simulink model "sgMdl_CAN_ParsingAndMapping"  (R2024b)
settings: Solver=FixedStepAuto  StartTime=0.0  StopTime=inf  RelTol=1e-3  EnableMultiTasking=on
model workspace (MAT data in the model file):
  mdlWSDbList = []
  mdlWSDbcList = "canConnectivityForVehicle.dbc"
undefined symbols (not defined in the file): DiscIntNeverNeededParam, Down, IO602, Pull
libraries: simulink x3, speedgoatlib_IO602_4 x1
Description:
  | CAN - Working with the DB Parser
settings Model: ModifiedByFormat=Speedgoat  Creator=Speedgoat  LastModifiedBy=Speedgoat
settings SolverCC: ConcurrentTasks=on  AlgebraicLoopSolver=TrustRegion  PositivePriorityOrder=on  InsertRTBMode=Never (minimum delay)
settings DataIOCC: SaveFormat=Array  SignalLoggingName=logsOut
settings OptimizationCC: BlockReduction=off  BooleanDataType=off  OptimizeBlockIOStorage=off  BufferReuse=off  ReuseModelBlockBuffer=off  GlobalBufferReuse=off  ExpressionFolding=off  LocalBlockOutputs=off  InitFltsAndDblsToZero=on  OptimizeDataStoreBuffers=off  BusAssignmentInplaceUpdate=off
settings DebuggingCC: SaveWithParameterizedLinksMsg=none  UnderspecifiedInitializationDetection=Classic  MergeDetectMultiDrivingBlocksExec=none  CheckExecutionContextPreStartOutputMsg=on  SignalResolutionControl=TryResolveAllWithWarning  TasksWithSamePriorityMsg=none  UnconnectedInputMsg=warning  UnconnectedOutputMsg=warning  UnconnectedLineMsg=warning  SFUnexpectedBacktrackingDiag=warning  SFNoUnconditionalDefaultTransitionDiag=warning  SFExecutionAtInitializationDiag=none  ArithmeticOperatorsInVariantConditions=warning
settings HardwareCC: ProdBitPerLong=64  ProdLongLongMode=on  ProdHWDeviceType=Intel->x86-64 (Linux 64)
settings ModelReferenceCC: EnableRefExpFcnMdlSchedulingChecks=on  PropagateSignalLabelsOutOfModel=off
settings SFSimCC: SimUseLocalCustomCode=off  SimTargetLang=C++
settings RTWCC: Description=Speedgoat Real-Time Target Machine  SystemTargetFile=speedgoat.tlc  TemplateMakefile=slrealtime_default_tmf  RTWUseLocalCustomCode=off  Toolchain=Simulink Real-Time Toolchain  BuildConfiguration=Faster Runs  TargetLang=C++  GPUComputeCapability=3.5  DLArmComputeVersion=19.05
settings CodeAppCC: StateflowObjectComments=on
settings SimulinkRealTimeTargetCC: SubcomponentCodeInterfacePackaging=Reusable function  MATLABClassNameForMDSCustomization=Simulink.SoftwareTarget.GRTCustomization  InstructionSetFMA=off  LogToMDFFile=off  SLRTFileLogMaxRuns=10
settings ConfigComp: CovMetricSettings=dw  CovSaveCumulativeToWorkspaceVar=on  CovSaveSingleToWorkspaceVar=on  CovExternalEMLEnable=off  CovSFcnEnable=off  CovBoundaryAbsTol=1.0e-5

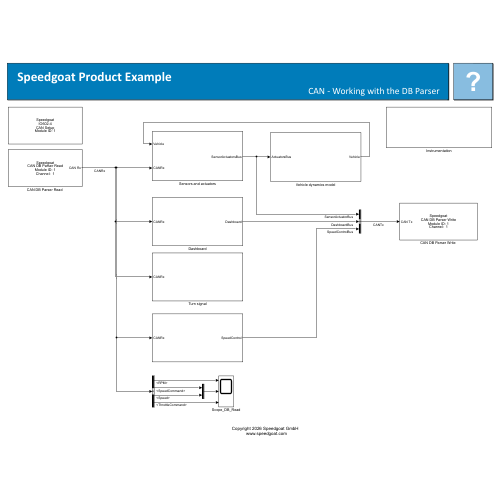
[thumbnail: Simulink's stored preview of the top-level diagram]
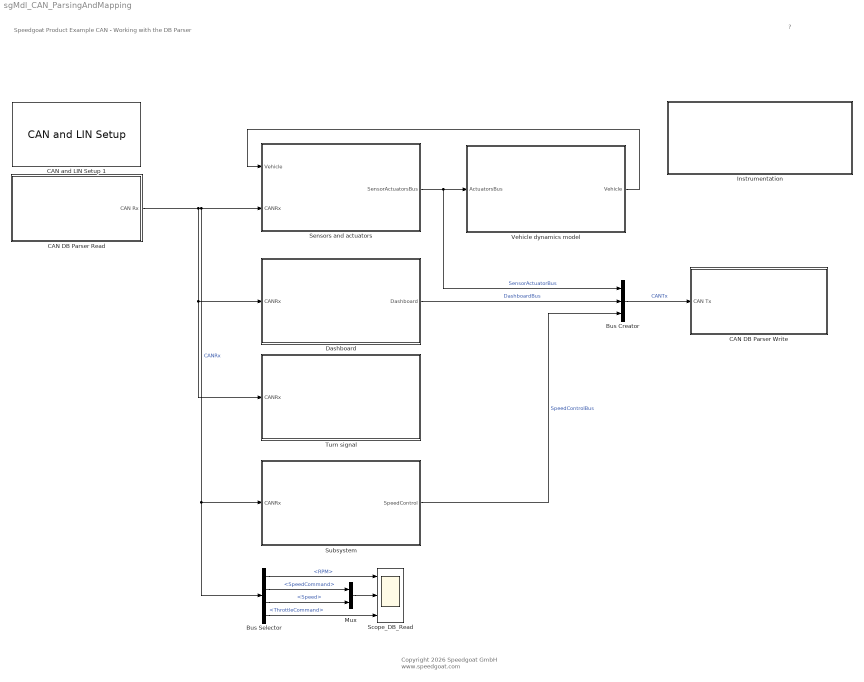
== system sgMdl_CAN_ParsingAndMapping ==
  note: Speedgoat Product Example
      | CAN - Working with the DB Parser
  note: ?
  note: Copyright 2026 Speedgoat GmbH
      |  www.speedgoat.com
  Bus Creator : BusCreator  Inputs=3
  Bus Selector : BusSelector  OutputSignals=ID2048_RPMMessage.RPM,ID1024_SpeedCommandMessage.SpeedCommand,ID256_SpeedMessage.Speed,ID96_ThrottleCommandMessage.ThrottleCommand
  "CAN DB Parser Read " : Subsystem
      settings: OpenFcn=sg_can.OpenFcnRead;
      mask Help: eval('sg.utils.help.show(''io_main/refentry_ref_can_ofa_parsing_read'');')
      mask Display: disp('Speedgoat\nCAN DB Parser Read\nModule ID: 1\nChannel:  1');
  "CAN DB Parser Write " : Subsystem
      settings: OpenFcn=sg_can.OpenFcnWrite;
      mask Help: eval('sg.utils.help.show(''io_main/refentry_ref_can_ofa_parsing_write'');')
      mask Display: disp('Speedgoat\nCAN DB Parser Write\nModule ID: 1\nChannel:  1');
  CAN and LIN Setup 1 : speedgoatlib_IO602_4/CAN and LIN Setup   moduleInitValues="[6022     1     1    -1    -1]"  id=1  moduleType=IO602-2  pciSlot=-1  canChn1=CAN (HS)  canChn2=CAN (HS)  canChn3=Disabled  canChn4=Disabled  linChn1=Disabled  linChn2=Disabled  canInitStructArray=[]  canTermStructArray=[]  gpioChnx=Disabled  canChn1InitValues="[2   2   8   1  16   3  19   2   2   5   2   0]"  arbBdrChn1=500 kBaud  clockDividerChn1=Enable  arbManBdrChn1=[8,1,16,3]  fdBdrChn1=5.0 MBaud  fdManBdrChn1=[2,2,5,2]  termResistor1=off  canChn2InitValues="[2   2   8   1  16   3  19   2   2   5   2   0]"  arbBdrChn2=500 kBaud  clockDividerChn2=Enable  arbManBdrChn2=[8,1,16,3]  fdBdrChn2=5.0 MBaud  fdManBdrChn2=[2,2,5,2]  termResistor2=off  canChn3InitValues="[1   0   2   8  31   8  19   2   2   5   2   0]"  arbBdrChn3=1.0 MBaud  clockDividerChn3=Enable  arbManBdrChn3=[2,8,31,8]  fdBdrChn3=5.0 MBaud  fdManBdrChn3=[2,2,5,2]  termResistor3=off  canChn4InitValues="[1   0   2   8  31   8  19   2   2   5   2   0]"  arbBdrChn4=1.0 MBaud  clockDividerChn4=Enable  arbManBdrChn4=[2,8,31,8]  fdBdrChn4=5.0 MBaud  fdManBdrChn4=[2,2,5,2]  termResistor4=off  linChn1InitValues="[0  9600]"  linBtrChn1=9600  linChn2InitValues="[0  9600]"  linBtrChn2=9600  doInitTermStruct="[0  5  0  0  0]"  parDoChannels=[1 2]  parDoVoltage=5  parDoInitValues=0  parDoReset=1  parNumOfDoS=0  parDiChannels=[3 4]  parDiVoltage=5  parDiPull=Pull-Down
      settings: LibrarySourceBlock=speedgoatlib_IO602_IO691/CAN and LIN Setup  SourceProductName=IO602-4
  Dashboard : Subsystem
  Instrumentation : Subsystem
  Mux : Mux  Inputs=2
  Scope_DB_Read : Scope  NumInputPorts=3
  Sensors and actuators : Subsystem
  Subsystem : Subsystem
  Turn signal : Subsystem
  Vehicle dynamics model : Subsystem
  wires:
  Vehicle dynamics model/1(Vehicle) -> Sensors and actuators/1(Vehicle)
  Sensors and actuators/1(SensorActuatorsBus) -> Bus Creator/1, Vehicle dynamics model/1(ActuatorsBus)  "SensorActuatorBus"
  Bus Creator/1 -> "CAN DB Parser Write "/1(CAN Tx)  "CANTx"
  Dashboard/1(Dashboard) -> Bus Creator/2  "DashboardBus"
  Subsystem/1(SpeedControl) -> Bus Creator/3  "SpeedControlBus"
  Mux/1 -> Scope_DB_Read/2
  Bus Selector/3 -> Mux/2  "<Speed>"
  Bus Selector/2 -> Mux/1  "<SpeedCommand>"
  "CAN DB Parser Read "/1(CAN Rx) -> Turn signal/1(CANRx), Dashboard/1(CANRx), Bus Selector/1, Subsystem/1(CANRx), Sensors and actuators/2(CANRx)  "CANRx"
  Bus Selector/1 -> Scope_DB_Read/1  "<RPM>"
  Bus Selector/4 -> Scope_DB_Read/3  "<ThrottleCommand>"

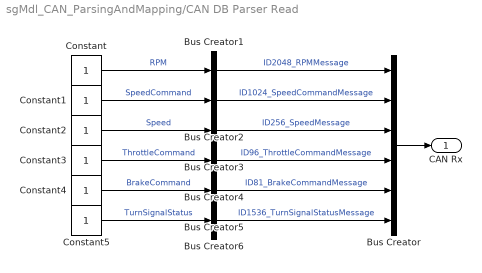
== system sgMdl_CAN_ParsingAndMapping/CAN DB Parser Read  ==
  Bus Creator : BusCreator  Inputs=6
  Bus Creator{1..6} (6 alike) : BusCreator  Inputs=1
  Constant{,1..5} (6 alike) : Constant  SampleTime=-1
  CAN Rx : Outport
  wires:
  Bus Creator4/1 -> Bus Creator/4  "ID96_ThrottleCommandMessage"
  Bus Creator1/1 -> Bus Creator/1  "ID2048_RPMMessage"
  Constant2/1 -> Bus Creator3/1  "Speed"
  Bus Creator2/1 -> Bus Creator/2  "ID1024_SpeedCommandMessage"
  Bus Creator5/1 -> Bus Creator/5  "ID81_BrakeCommandMessage"
  Constant5/1 -> Bus Creator6/1  "TurnSignalStatus"
  Constant4/1 -> Bus Creator5/1  "BrakeCommand"
  Constant1/1 -> Bus Creator2/1  "SpeedCommand"
  Constant3/1 -> Bus Creator4/1  "ThrottleCommand"
  Bus Creator/1 -> CAN Rx/1
  Bus Creator3/1 -> Bus Creator/3  "ID256_SpeedMessage"
  Constant/1 -> Bus Creator1/1  "RPM"
  Bus Creator6/1 -> Bus Creator/6  "ID1536_TurnSignalStatusMessage"

== system sgMdl_CAN_ParsingAndMapping/CAN DB Parser Write  ==
  CAN Tx : Inport
  Terminator : Terminator
  wires:
  CAN Tx/1 -> Terminator/1

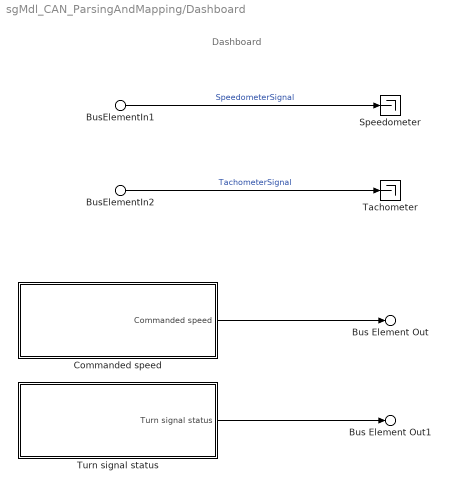
== system sgMdl_CAN_ParsingAndMapping/Dashboard ==
  note: Dashboard
  BusElementIn1 : Inport  PortName=CANRx  Element=ID256_SpeedMessage.Speed
  BusElementIn2 : Inport  PortName=CANRx  Element=ID2048_RPMMessage.RPM
  Commanded speed : Subsystem
  Speedometer : Terminator
  Tachometer : Terminator
  Turn signal status : Subsystem
  Bus Element Out : Outport  PortName=Dashboard  Element=SpeedComand
  Bus Element Out1 : Outport  PortName=Dashboard  Element=TurnSignalStatus
  wires:
  BusElementIn2/1 -> Tachometer/1  "TachometerSignal"
  BusElementIn1/1 -> Speedometer/1  "SpeedometerSignal"
  Commanded speed/1(Commanded speed) -> Bus Element Out/1
  Turn signal status/1(Turn signal status) -> Bus Element Out1/1

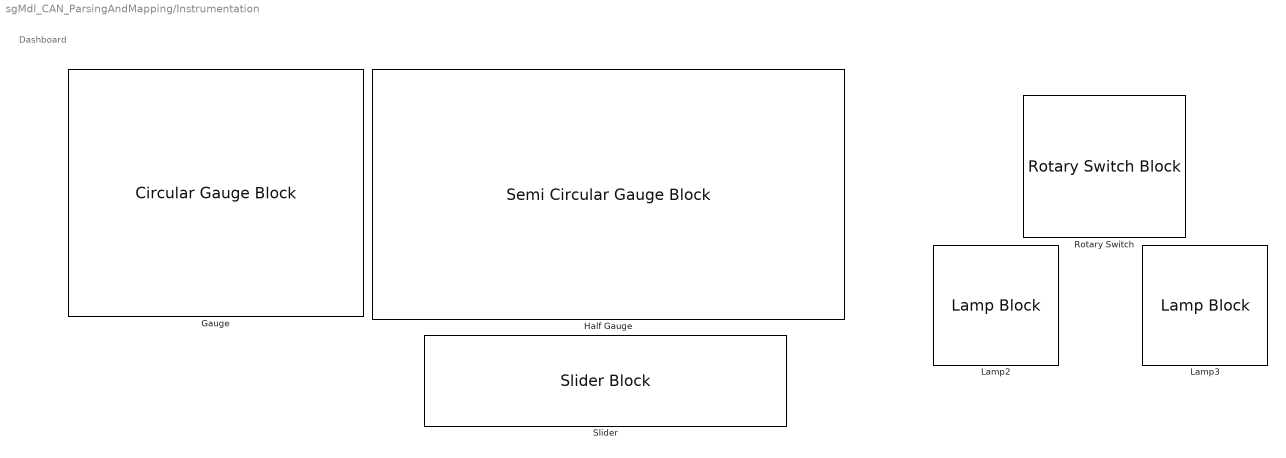
== system sgMdl_CAN_ParsingAndMapping/Instrumentation ==
  note: Dashboard
  Gauge : CircularGaugeBlock  TickInterval=10
  Half Gauge : SemiCircularGaugeBlock  ScaleMax=9000  TickInterval=1000
  Lamp2 : LampBlock
  Lamp3 : LampBlock
  Rotary Switch : RotarySwitchBlock
      settings: Values={{'Left', 'Off', 'Right'}, [1 2 3]}
  Slider : SliderBlock

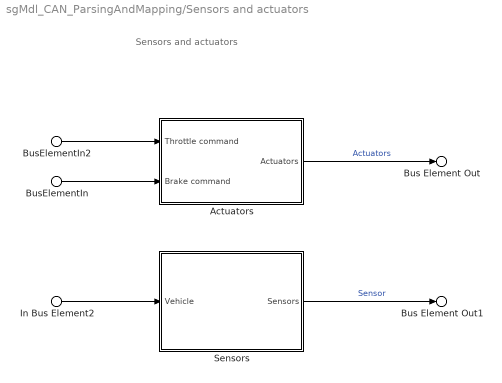
== system sgMdl_CAN_ParsingAndMapping/Sensors and actuators ==
  note: Sensors and actuators
  In Bus Element2 : Inport  PortName=Vehicle
  BusElementIn2 : Inport  Port=2  PortName=CANRx  Element=ID96_ThrottleCommandMessage.ThrottleCommand
  BusElementIn : Inport  Port=2  PortName=CANRx  Element=ID81_BrakeCommandMessage.BrakeCommand
  Actuators : Subsystem
  Sensors : Subsystem
  Bus Element Out : Outport  PortName=SensorActuatorsBus  Element=Actuators
  Bus Element Out1 : Outport  PortName=SensorActuatorsBus  Element=Sensors
  wires:
  Actuators/1(Actuators) -> Bus Element Out/1  "Actuators"
  Sensors/1(Sensors) -> Bus Element Out1/1  "Sensor"
  BusElementIn2/1 -> Actuators/1(Throttle command)
  BusElementIn/1 -> Actuators/2(Brake command)
  In Bus Element2/1 -> Sensors/1(Vehicle)

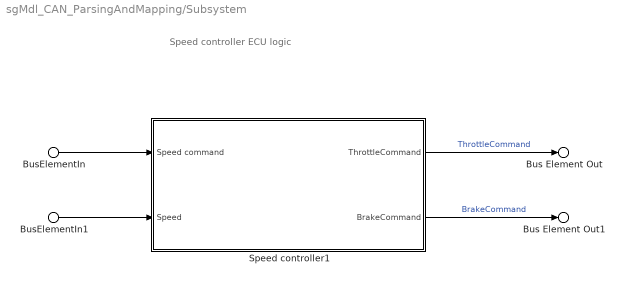
== system sgMdl_CAN_ParsingAndMapping/Subsystem ==
  note: Speed controller ECU logic
  BusElementIn : Inport  PortName=CANRx  Element=ID1024_SpeedCommandMessage.SpeedCommand
  BusElementIn1 : Inport  PortName=CANRx  Element=ID256_SpeedMessage.Speed
  Speed controller1 : Subsystem
  Bus Element Out : Outport  PortName=SpeedControl  Element=ThrottleCommand
  Bus Element Out1 : Outport  PortName=SpeedControl  Element=BrakeCommand
  wires:
  BusElementIn/1 -> Speed controller1/1(Speed command)
  BusElementIn1/1 -> Speed controller1/2(Speed)
  Speed controller1/1(ThrottleCommand) -> Bus Element Out/1  "ThrottleCommand"
  Speed controller1/2(BrakeCommand) -> Bus Element Out1/1  "BrakeCommand"

== system sgMdl_CAN_ParsingAndMapping/Turn signal ==
  note: Turn signal ECU logic
  BusElementIn : Inport  PortName=CANRx  Element=ID1536_TurnSignalStatusMessage.TurnSignalStatus
  Left turn signal : Terminator
  Right turn signal : Terminator
  Turn signal logic : Subsystem
  wires:
  Turn signal logic/1(Left turn signal interface) -> Left turn signal/1  "LeftTurnSignal"
  Turn signal logic/2(Right turn signal interface) -> Right turn signal/1  "RightTurnSignal"
  BusElementIn/1 -> Turn signal logic/1(Turn signal status)

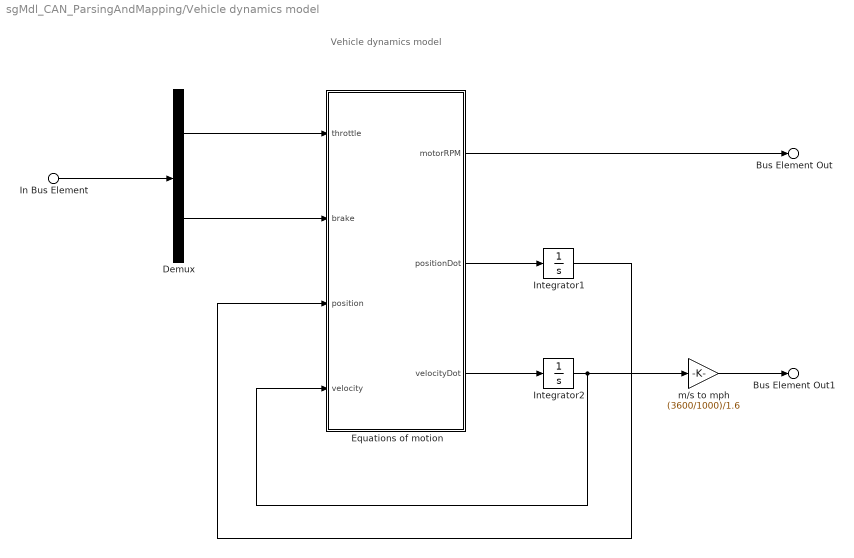
== system sgMdl_CAN_ParsingAndMapping/Vehicle dynamics model ==
  note: Vehicle dynamics model
  In Bus Element : Inport  PortName=ActuatorsBus  Element=Actuators.Control
  Demux : Demux  Outputs=2
  Equations of motion : Subsystem
  Integrator1 : Integrator
  Integrator2 : Integrator
  m/s to mph : Gain  Gain=(3600/1000)/1.6
  Bus Element Out : Outport  PortName=Vehicle  Element=motorRPM
  Bus Element Out1 : Outport  PortName=Vehicle  Element=Velocity
  wires:
  Demux/1 -> Equations of motion/1(throttle)
  Equations of motion/2(positionDot) -> Integrator1/1
  Equations of motion/3(velocityDot) -> Integrator2/1
  Integrator2/1 -> Equations of motion/4(velocity), m/s to mph/1
  Integrator1/1 -> Equations of motion/3(position)
  Demux/2 -> Equations of motion/2(brake)
  Equations of motion/1(motorRPM) -> Bus Element Out/1
  In Bus Element/1 -> Demux/1
  m/s to mph/1 -> Bus Element Out1/1

== system sgMdl_CAN_ParsingAndMapping/Dashboard/Commanded speed ==
  note: Commanded speed
  Speed command : Constant  Value=33.01438748428551  OutDataTypeStr=double  SampleTime=Inf
  Zero-Order Hold : ZeroOrderHold  SampleTime=-1
  Commanded speed : Outport  VectorParamsAs1DForOutWhenUnconnected=off
  wires:
  Speed command/1 -> Zero-Order Hold/1
  Zero-Order Hold/1 -> Commanded speed/1

== system sgMdl_CAN_ParsingAndMapping/Dashboard/Turn signal status ==
  note: Turn signal status
  Turn signal : Constant  Value=2  OutDataTypeStr=double
  Zero-Order Hold : ZeroOrderHold  SampleTime=-1
  Turn signal status : Outport  VectorParamsAs1DForOutWhenUnconnected=off
  wires:
  Turn signal/1 -> Zero-Order Hold/1
  Zero-Order Hold/1 -> Turn signal status/1

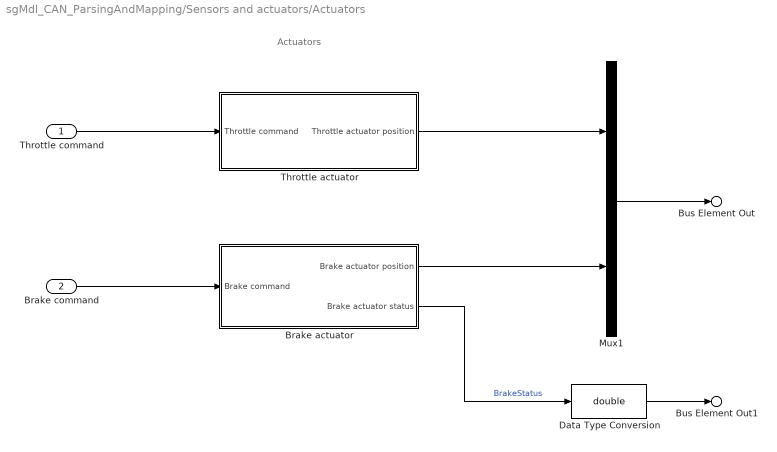
== system sgMdl_CAN_ParsingAndMapping/Sensors and actuators/Actuators ==
  note: Actuators
  Throttle command : Inport
  Brake command : Inport  Port=2
  Brake actuator : Subsystem
  Data Type Conversion : DataTypeConversion  OutDataTypeStr=double  SaturateOnIntegerOverflow=off  RndMeth=Floor
  Mux1 : Mux  Inputs=2
  Throttle actuator : Subsystem
  Bus Element Out : Outport  PortName=Actuators  Element=Control
  Bus Element Out1 : Outport  PortName=Actuators  Element=BrakeStatus
  wires:
  Brake actuator/1(Brake actuator position) -> Mux1/2
  Throttle actuator/1(Throttle actuator position) -> Mux1/1
  Brake command/1 -> Brake actuator/1(Brake command)
  Throttle command/1 -> Throttle actuator/1(Throttle command)
  Data Type Conversion/1 -> Bus Element Out1/1
  Brake actuator/2(Brake actuator status) -> Data Type Conversion/1  "BrakeStatus"
  Mux1/1 -> Bus Element Out/1

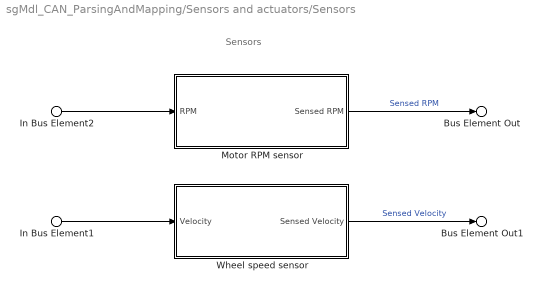
== system sgMdl_CAN_ParsingAndMapping/Sensors and actuators/Sensors ==
  note: Sensors
  In Bus Element2 : Inport  PortName=Vehicle  Element=motorRPM
  In Bus Element1 : Inport  PortName=Vehicle  Element=Velocity
  Motor RPM sensor : Subsystem
  Wheel speed sensor : Subsystem
  Bus Element Out : Outport  PortName=Sensors  Element=RPM
  Bus Element Out1 : Outport  PortName=Sensors  Element=Speed
  wires:
  In Bus Element2/1 -> Motor RPM sensor/1(RPM)
  In Bus Element1/1 -> Wheel speed sensor/1(Velocity)
  Wheel speed sensor/1(Sensed Velocity) -> Bus Element Out1/1  "Sensed Velocity"
  Motor RPM sensor/1(Sensed RPM) -> Bus Element Out/1  "Sensed RPM"

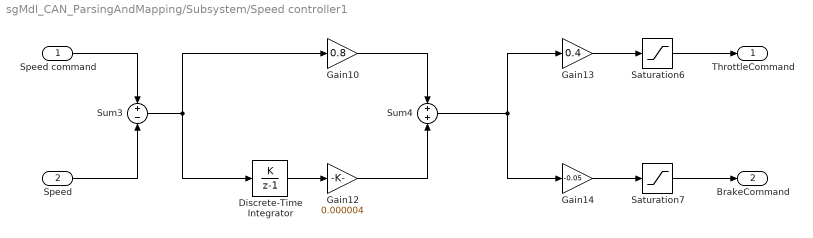
== system sgMdl_CAN_ParsingAndMapping/Subsystem/Speed controller1 ==
  Speed command : Inport
  Speed : Inport  Port=2
  Discrete-Time Integrator : DiscreteIntegrator  IntegratorMethod=Accumulation: Forward Euler  SampleTime=-1  ICPrevOutput=DiscIntNeverNeededParam  ICPrevScaledInput=DiscIntNeverNeededParam
  Gain10 : Gain  Gain=0.8
  Gain12 : Gain  Gain=0.000004
  Gain13 : Gain  Gain=0.4
  Gain14 : Gain  Gain=-0.05
  Saturation6 : Saturate  UpperLimit=1  LowerLimit=0
  Saturation7 : Saturate  UpperLimit=1  LowerLimit=0
  Sum3 : Sum  Inputs=+|-
  Sum4 : Sum  Inputs=+|+
  ThrottleCommand : Outport  VectorParamsAs1DForOutWhenUnconnected=off
  BrakeCommand : Outport  Port=2  VectorParamsAs1DForOutWhenUnconnected=off
  wires:
  Saturation7/1 -> BrakeCommand/1
  Saturation6/1 -> ThrottleCommand/1
  Speed command/1 -> Sum3/1
  Speed/1 -> Sum3/2
  Sum3/1 -> Discrete-Time Integrator/1, Gain10/1
  Discrete-Time Integrator/1 -> Gain12/1
  Gain10/1 -> Sum4/1
  Sum4/1 -> Gain14/1, Gain13/1
  Gain14/1 -> Saturation7/1
  Gain13/1 -> Saturation6/1
  Gain12/1 -> Sum4/2

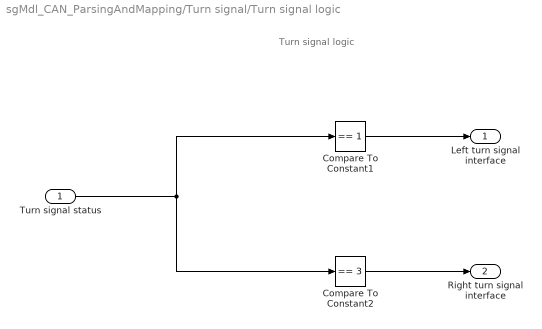
== system sgMdl_CAN_ParsingAndMapping/Turn signal/Turn signal logic ==
  note: Turn signal logic
  Turn signal status : Inport
  Compare To Constant1 : simulink/Logic and Bit Operations/Compare To Constant  relop===  const=1  OutDataTypeStr=boolean
  Compare To Constant2 : simulink/Logic and Bit Operations/Compare To Constant  relop===  const=3  OutDataTypeStr=boolean
  Left turn signal interface : Outport  VectorParamsAs1DForOutWhenUnconnected=off
  Right turn signal interface : Outport  Port=2  VectorParamsAs1DForOutWhenUnconnected=off
  wires:
  Turn signal status/1 -> Compare To Constant2/1, Compare To Constant1/1
  Compare To Constant2/1 -> Right turn signal interface/1
  Compare To Constant1/1 -> Left turn signal interface/1

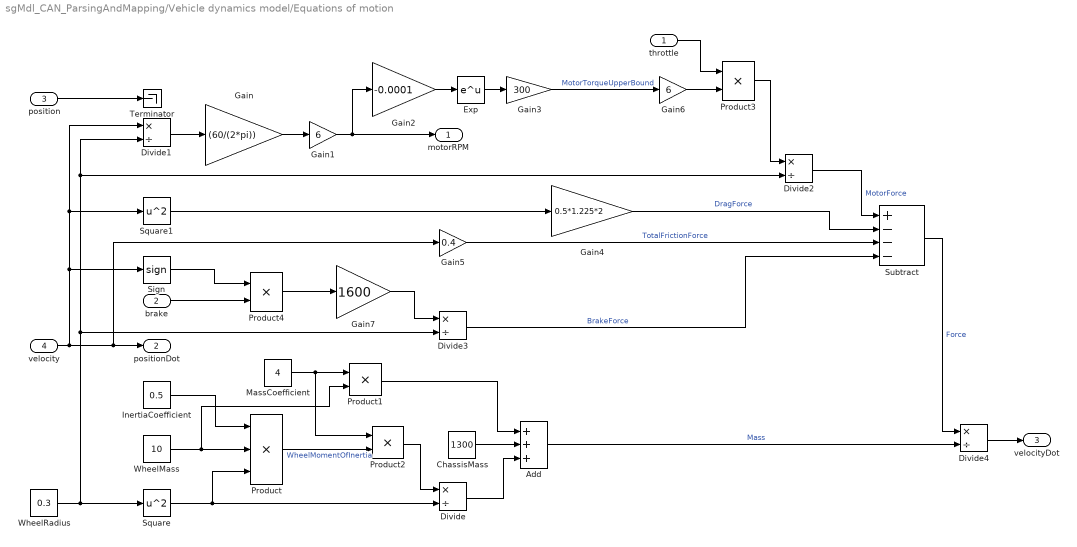
== system sgMdl_CAN_ParsingAndMapping/Vehicle dynamics model/Equations of motion ==
  throttle : Inport
  brake : Inport  Port=2
  position : Inport  Port=3
  velocity : Inport  Port=4
  Add : Sum  Inputs=+++
  ChassisMass : Constant  Value=1300
  Divide{,1..4} (5 alike) : Product  Inputs=*/
  Exp : Math
  Gain : Gain  Gain=(60/(2*pi))
  Gain1 : Gain  Gain=6
  Gain2 : Gain  Gain=-0.0001
  Gain3 : Gain  Gain=300
  Gain4 : Gain  Gain=0.5*1.225*2
  Gain5 : Gain  Gain=0.4
  Gain6 : Gain  Gain=6
  Gain7 : Gain  Gain=1600
  InertiaCoefficient : Constant  Value=0.5
  MassCoefficient : Constant  Value=4
  Product : Product  Inputs=3
  Product{1..4} (4 alike) : Product
  Sign : Signum
  Square : Math  Operator=square
  Square1 : Math  Operator=square
  Subtract : Sum  Inputs=+---
  Terminator : Terminator
  WheelMass : Constant  Value=10
  WheelRadius : Constant  Value=0.3
  motorRPM : Outport
  positionDot : Outport  Port=2
  velocityDot : Outport  Port=3
  wires:
  Square1/1 -> Gain4/1
  position/1 -> Terminator/1
  brake/1 -> Product4/2
  velocity/1 -> Gain5/1, positionDot/1, Square1/1, Divide1/1, Sign/1
  InertiaCoefficient/1 -> Product/1
  WheelRadius/1 -> Divide1/2, Divide2/2, Divide3/2, Square/1
  Gain6/1 -> Product3/2
  Divide1/1 -> Gain/1
  Gain3/1 -> Gain6/1  "MotorTorqueUpperBound"
  Sign/1 -> Product4/1
  WheelMass/1 -> Product1/2, Product/2
  Gain4/1 -> Subtract/2  "DragForce"
  Square/1 -> Divide/2, Product/3
  Divide/1 -> Add/3
  Gain/1 -> Gain1/1
  Product4/1 -> Gain7/1
  ChassisMass/1 -> Add/2
  MassCoefficient/1 -> Product1/1, Product2/1
  Product/1 -> Product2/2  "WheelMomentOfInertia"
  Exp/1 -> Gain3/1
  Gain1/1 -> motorRPM/1, Gain2/1
  Gain7/1 -> Divide3/1
  Product1/1 -> Add/1
  Gain5/1 -> Subtract/3  "TotalFrictionForce"
  Product2/1 -> Divide/1
  Gain2/1 -> Exp/1
  Divide3/1 -> Subtract/4  "BrakeForce"
  Add/1 -> Divide4/2  "Mass"
  throttle/1 -> Product3/1
  Product3/1 -> Divide2/1
  Divide2/1 -> Subtract/1  "MotorForce"
  Subtract/1 -> Divide4/1  "Force"
  Divide4/1 -> velocityDot/1

== system sgMdl_CAN_ParsingAndMapping/Sensors and actuators/Actuators/Brake actuator ==
  note: Brake actuator
  Brake command : Inport
  Brake actuator : TransferFcn  Denominator=[0.1 1]
  Brake status sensor : Subsystem
  Brake actuator position : Outport  VectorParamsAs1DForOutWhenUnconnected=off
  Brake actuator status : Outport  Port=2  VectorParamsAs1DForOutWhenUnconnected=off
  wires:
  Brake status sensor/1(Brake status) -> Brake actuator status/1
  Brake command/1 -> Brake actuator/1
  Brake actuator/1 -> Brake actuator position/1, Brake status sensor/1(Brake actuator position)

== system sgMdl_CAN_ParsingAndMapping/Sensors and actuators/Actuators/Throttle actuator ==
  note: Throttle actuator
  Throttle command : Inport
  Throttle actuator : TransferFcn  Denominator=[0.1 1]
  Throttle actuator position : Outport  VectorParamsAs1DForOutWhenUnconnected=off
  wires:
  Throttle command/1 -> Throttle actuator/1
  Throttle actuator/1 -> Throttle actuator position/1

== system sgMdl_CAN_ParsingAndMapping/Sensors and actuators/Sensors/Motor RPM sensor ==
  note: Motor RPM sensor
  RPM : Inport
  Zero-Order Hold : ZeroOrderHold  SampleTime=.01
  Sensed RPM : Outport  VectorParamsAs1DForOutWhenUnconnected=off
  wires:
  Zero-Order Hold/1 -> Sensed RPM/1
  RPM/1 -> Zero-Order Hold/1

== system sgMdl_CAN_ParsingAndMapping/Sensors and actuators/Sensors/Wheel speed sensor ==
  note: Wheel speed sensor
  Velocity : Inport
  Zero-Order Hold : ZeroOrderHold  SampleTime=.01
  Sensed Velocity : Outport  VectorParamsAs1DForOutWhenUnconnected=off
  wires:
  Zero-Order Hold/1 -> Sensed Velocity/1
  Velocity/1 -> Zero-Order Hold/1

== system sgMdl_CAN_ParsingAndMapping/Sensors and actuators/Actuators/Brake actuator/Brake status sensor ==
  note: Brake status sensor
  Brake actuator position : Inport
  Compare To Constant : simulink/Logic and Bit Operations/Compare To Constant  relop=>  const=0.01  OutDataTypeStr=boolean
  Zero-Order Hold : ZeroOrderHold  SampleTime=0.01
  Brake status : Outport  VectorParamsAs1DForOutWhenUnconnected=off
  wires:
  Zero-Order Hold/1 -> Brake status/1
  Brake actuator position/1 -> Compare To Constant/1
  Compare To Constant/1 -> Zero-Order Hold/1
